simulink model "rodoautoattempt"  (R2015b)
settings: Solver=FixedStepAuto  StartTime=0.0  StopTime=1  FixedStep=0.001  RelTol=1e-3
values from neighbouring files (symbols this model uses):
  C = [1 0]    [ssmodel.m]    (also in ssmodel2.m = [1 0 0])
  Ga = [E G]    [ssmodel2.m]
  P = dare(phi_aug, gamma_aug, Q, R)    [ecs.m]    (also in ssmodel2.m = [eval(p1sol) eval(p2sol) eval(p3sol); eval(p4sol) eval(p5sol)
  pol1 = 0.5    [ssmodel2.m]
  pol2 = 0.55    [ssmodel2.m]
undefined symbols (not defined in the file or in its folder): Ad2, Bd2, Cd2, Dd2
settings Model: Creator=ADMIN  LastModifiedBy=ADMIN

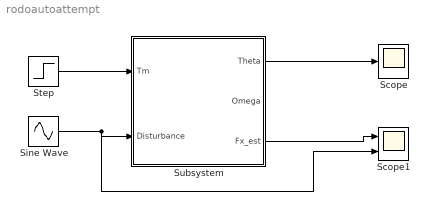
== system rodoautoattempt ==
  Scope : Scope
  Scope1 : Scope  NumInputPorts=2
  Sine Wave : Sin  Frequency=50
  Step : Step  Time=0.01
  Subsystem : Subsystem  InitFcn=|
      | rw = 0.5;
      | Iw = 12.5;
      | pol1 = 0.5;
      | pol2 = 0.55;
      | A = [0 1 0; 0 0 -rw/Iw; 0 0 0];
      | B = [0 ; 1/Iw ; 0];
      | C = [1 0 0];
      | Do = 0;
      | Ts = 0.001;
      | 
      | systa = ss(A,B,C,Do);
      | systaa = c2d(systa, Ts);
      | Ad = systaa.a;
      | Bd = systaa.b;
      | Cd = systaa.c;
      | 
      | A2 = [ 0 1; 0 0 ];
      | B2 = [ 0 0; 1/Iw -rw/Iw];
      | C2 = [1 0];
      | D2 = [0 0];
      | 
      | sys2 = ss(A2,B2,C2,D2);
      | sysdis2 = c2d(sys2, Ts);
      | Ad2 = sysdis2.a;
      | Bd2 = sysdis2.b;
      | Cd2 = sysdis2.c;
      | Dd2 = sysdis2.d;
      | 
      | syms p1 p2 p3 p4 p5 p6; %unknowns
      | P = [p1 p2 p3; p4 p5 p6];
      | D = [0.5 0 ; 0 0.55];
      | G = [5 ; 10];%observer gain
      | [p1sol, p2sol, p3sol, p4sol, p5sol, p6sol] = solve(P*Ad - D*P == G*Cd);
      | P = [eval(p1sol) eval(p2sol) eval(p3sol); eval(p4sol) eval(p5sol) eval(p6sol)];
      | 
      | E = P*Bd;
      | 
      | Ga = [E G];
  wires:
  Sine Wave/1 -> Scope1/2, Subsystem/2(Disturbance)
  Step/1 -> Subsystem/1(Tm)
  Subsystem/3(Fx_est) -> Scope1/1
  Subsystem/1(Theta) -> Scope/1

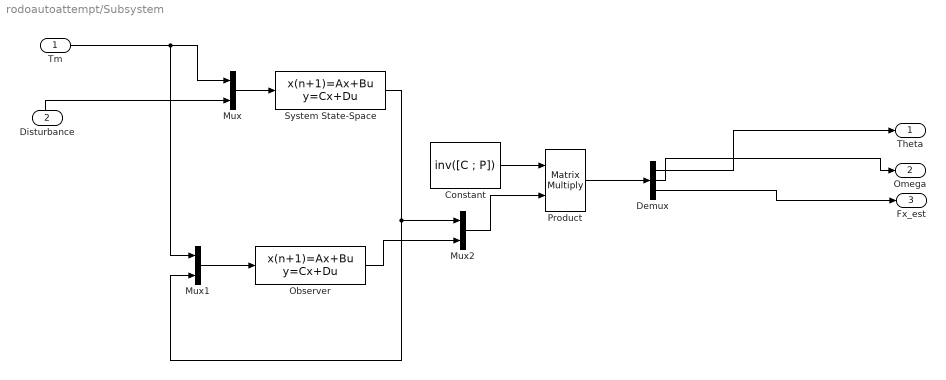
== system rodoautoattempt/Subsystem ==
  Tm : Inport
  Disturbance : Inport  Port=2
  Constant : Constant  Value=inv([C ; P])
  Demux : Demux  Outputs=3
  Mux : Mux  Inputs=2
  Mux1 : Mux  Inputs=2
  Mux2 : Mux  Inputs=2
  Observer : DiscreteStateSpace  A=[pol1 0 ; 0 pol2]  B=Ga  C=[1 0; 0 1]  D=[0 0; 0 0]  SampleTime=-1
  Product : Product  Multiplication=Matrix(*)
  System State-Space : DiscreteStateSpace  A=Ad2  B=Bd2  C=Cd2  D=Dd2  SampleTime=-1
  Theta : Outport
  Omega : Outport  Port=2
  Fx_est : Outport  Port=3
  wires:
  Mux2/1 -> Product/2
  Demux/3 -> Fx_est/1
  Product/1 -> Demux/1
  Constant/1 -> Product/1
  Tm/1 -> Mux1/1, Mux/1
  Mux/1 -> System State-Space/1
  System State-Space/1 -> Mux2/1, Mux1/2
  Mux1/1 -> Observer/1
  Observer/1 -> Mux2/2
  Disturbance/1 -> Mux/2
  Demux/1 -> Theta/1
  Demux/2 -> Omega/1
